simulink model "Optical_Movement_Detection_PAR"  (Simulink 7.5)
settings: Solver=ode45  StartTime=0.0  StopTime=inf  RelTol=1e-3
values from neighbouring files (symbols this model uses):
  D = 1    [Copter_Animation.m]
undefined symbols (not defined in the file or in its folder): Bottom, fspecial, Low, Rec, SDTV, sigbuilder_block
libraries: simulink x10, dspobslib x5, vipgeotforms x3, dspmtrx3 x2, vipanalysis x2, viptextngfix x2, vipsnks x2, dspsigops x2, vipconversions x1, dspswit3 x1, vipsrcs x1, dspstat3 x1
(part 2 of 2)

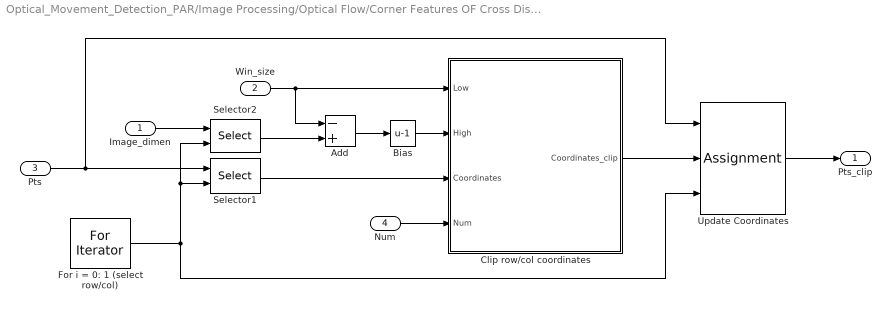
== system Optical_Movement_Detection_PAR/Image Processing/Optical Flow/Corner Features OF Cross Display/Corner Features OF/Corner Matching/Calculate Features/Clip Point Coordinates ==
  Image_dimen : Inport  OutDataType=sfix(16)  OutScaling=2^0
  Win_size : Inport  Port=2  OutDataType=sfix(16)  OutScaling=2^0
  Pts : Inport  Port=3
  Num : Inport  Port=4
  Add : Sum  Inputs=-+  OutDataType=sfix(16)  OutScaling=2^-10
  Bias : Bias  Bias=-1
  Clip row/col coordinates : Subsystem
  For i = 0: 1 (select row/col) : ForIterator  IterationLimit=2  IndexMode=Zero-based
  Selector1 : Selector  NumberOfDimensions=2  IndexMode=Zero-based  InputPortWidth=3  IndexOptions=Index vector (port),Select all  Indices=[1 3],1  OutputSizes=9,9
  Selector2 : Selector  IndexMode=Zero-based  InputPortWidth=2  IndexOptions=Index vector (port)  Indices=[1 3]  OutputSizes=9
  Update Coordinates : Assignment  NumberOfDimensions=2  IndexMode=Zero-based  IndexOptions=Index vector (port),Assign all  Indices=1,1  OutputSizes=81,50
  Pts_clip : Outport  OutDataType=sfix(16)  OutScaling=2^0
  wires:
  Selector2/1 -> Add/2
  For i = 0: 1 (select row/col)/1 -> Selector1/2, Selector2/2, Update Coordinates/3
  Clip row/col coordinates/1(Coordinates_clip) -> Update Coordinates/2
  Bias/1 -> Clip row/col coordinates/2(High)
  Update Coordinates/1 -> Pts_clip/1
  Num/1 -> Clip row/col coordinates/4(Num)
  Selector1/1 -> Clip row/col coordinates/3(Coordinates)
  Win_size/1 -> Add/1, Clip row/col coordinates/1(Low)
  Add/1 -> Bias/1
  Image_dimen/1 -> Selector2/1
  Pts/1 -> Update Coordinates/1, Selector1/1

== system Optical_Movement_Detection_PAR/Image Processing/Optical Flow/Corner Features OF Cross Display/Corner Features OF/Corner Matching/Calculate Distances/For Iterator Subsystem/For Iterator Subsystem ==
  F1 : Inport  OutDataType=sfix(16)  OutScaling=2^0
  N1 : Inport  Port=2  OutDataType=sfix(16)  OutScaling=2^0
  f2 : Inport  Port=3  OutDataType=sfix(16)  OutScaling=2^0
  Distance between two feature vectors : Subsystem
  For Iterator : ForIterator  IterationSource=external  IndexMode=Zero-based
  Select feature  for 1 corner : Selector  NumberOfDimensions=2  IndexMode=Zero-based  InputPortWidth=2  IndexOptions=Select all,Index vector (port)  Indices=0,1  OutputSizes=1,1
  Update feature  for a corner : Assignment  NumberOfDimensions=2  IndexMode=Zero-based  OutputInitialize=Specify size for each dimension in table  IndexOptions=Index vector (port),Assign all  Indices=1,1  OutputSizes=maxNum,1
  Dis : Outport  OutDataType=sfix(16)  OutScaling=2^0
  wires:
  Select feature  for 1 corner/1 -> Distance between two feature vectors/1(f1)
  f2/1 -> Distance between two feature vectors/2(f2)
  Update feature  for a corner/1 -> Dis/1
  F1/1 -> Select feature  for 1 corner/1
  For Iterator/1 -> Select feature  for 1 corner/2, Update feature  for a corner/2
  N1/1 -> For Iterator/1
  Distance between two feature vectors/1(dis) -> Update feature  for a corner/1

== system Optical_Movement_Detection_PAR/Image Processing/Optical Flow/Corner Features OF Cross Display/Corner Features OF/Corner Matching/Calculate Features/Clip Point Coordinates/Clip row/col coordinates ==
  Low : Inport  OutDataType=sfix(16)  OutScaling=2^0
  High : Inport  Port=2  OutDataType=sfix(16)  OutScaling=2^0
  Coordinates : Inport  Port=3
  Num : Inport  Port=4  OutDataType=sfix(16)  OutScaling=2^0
  Clip a Coordinate : Subsystem
  For Iterator : ForIterator  IterationSource=external  IterationLimit=2  IndexMode=Zero-based
  Select Coordinate of a Point : Selector  NumberOfDimensions=2  IndexMode=Zero-based  InputPortWidth=3  IndexOptions=Select all,Index vector (port)  Indices=[1 3],1  OutputSizes=9,1
  Update Feature  for a Corner : Assignment  NumberOfDimensions=2  IndexMode=Zero-based  IndexOptions=Assign all,Index vector (port)  Indices=1,1  OutputSizes=81,50
  Coordinates_clip : Outport  OutDataType=sfix(16)  OutScaling=2^0
  wires:
  Clip a Coordinate/1(Coordinate_clip) -> Update Feature  for a Corner/2
  Update Feature  for a Corner/1 -> Coordinates_clip/1
  High/1 -> Clip a Coordinate/2(High)
  Low/1 -> Clip a Coordinate/1(Low)
  Select Coordinate of a Point/1 -> Clip a Coordinate/3(Coordinate)
  Num/1 -> For Iterator/1
  Coordinates/1 -> Update Feature  for a Corner/1, Select Coordinate of a Point/1
  For Iterator/1 -> Select Coordinate of a Point/2, Update Feature  for a Corner/3

== system Optical_Movement_Detection_PAR/Image Processing/Optical Flow/Corner Features OF Cross Display/Corner Features OF/Corner Matching/Calculate Distances/For Iterator Subsystem/For Iterator Subsystem/Distance between two feature vectors ==
  f1 : Inport  OutDataType=sfix(16)  OutScaling=2^0
  f2 : Inport  Port=2  OutDataType=sfix(16)  OutScaling=2^0
  Abs : Abs  OutDataType=sfix(16)  OutScaling=2^0
  Add : Sum  Inputs=+-  OutDataType=sfix(16)  OutScaling=2^-10
  Sum of Elements : Sum  Inputs=+  OutDataType=sfix(16)  OutScaling=2^-10
  dis : Outport  OutDataType=sfix(16)  OutScaling=2^0
  wires:
  Sum of Elements/1 -> dis/1
  Abs/1 -> Sum of Elements/1
  Add/1 -> Abs/1
  f2/1 -> Add/2
  f1/1 -> Add/1

== system Optical_Movement_Detection_PAR/Image Processing/Optical Flow/Corner Features OF Cross Display/Corner Features OF/Corner Matching/Calculate Features/Clip Point Coordinates/Clip row/col coordinates/Clip a Coordinate ==
  Low : Inport  OutDataType=sfix(16)  OutScaling=2^0
  High : Inport  Port=2  OutDataType=sfix(16)  OutScaling=2^0
  Coordinate : Inport  Port=3  OutDataType=sfix(16)  OutScaling=2^0
  MinMax1 : MinMax  Function=max  Inputs=2  OutDataType=sfix(16)  OutScaling=2^0
  MinMax2 : MinMax  Inputs=2  OutDataType=sfix(16)  OutScaling=2^0
  Coordinate_clip : Outport  OutDataType=sfix(16)  OutScaling=2^0
  wires:
  MinMax2/1 -> Coordinate_clip/1
  High/1 -> MinMax2/2
  MinMax1/1 -> MinMax2/1
  Low/1 -> MinMax1/2
  Coordinate/1 -> MinMax1/1

== matlab function Image Processing/Optical Flow/Block Matching OF Cross Display/Optical Flow Segmentation in Sectors/Optical Flow Lines1 ==
  data: vel_Values input double; Cam_Img_Dim input double; vel_Lines output double; Omega_avg output double; scaleFactor parameter double size=1
function [vel_Lines, Omega_avg]=OpticalFlowLines(vel_Values, Cam_Img_Dim,scaleFactor) 

% Generates the coordinate points of optical flow lines

persistent first_time;
persistent X;
persistent Y;
persistent RV;
persistent CV;

%persistent Max_Vec_Length;

persistent Origin_Re;
persistent Origin_Im;

persistent Sec_1_Cnt;
persistent Sec_2_Cnt;
persistent Sec_3_Cnt;
persistent Sec_4_Cnt;

persistent Sec_1;
persistent Sec_2;
persistent Sec_3;
persistent Sec_4;

persistent R;
persistent C;
persistent Test_mat;
persistent med_vel_val;

%med_vel_val=median(vel_Values);
%[R C] = size(med_vel_val);
if isempty(first_time)
    first_time     = 1;
    Origin_Re = Cam_Img_Dim(1)/2%double(176);
    [R C] = size(vel_Values)
    Origin_Im = Cam_Img_Dim(2)/2%double(144);
end

Sec_1 = double(0);
Sec_2 = double(0);
Sec_3 = double(0);
Sec_4 = double(0);

Sec_1_Cnt = 1;
Sec_2_Cnt = 1;
Sec_3_Cnt = 1;
Sec_4_Cnt = 1;

%sectors
%       ^Im
%       |         
%   4   |  1
%-------------->Re
%   3   |  2
%       |

% for i=1:R
%     for k=1:C
%       j=vel_Values(i,k);
%     if(real(j)>=0) % Sec_1 or Sec_2
%         if(imag(j)>=0) %Sec_1
%             Sec_1_Cnt=Sec_1_Cnt+1;
%             Sec_1=Sec_1+double(abs(j))
%         else           %Sec_2
%             Sec_2_Cnt=Sec_2_Cnt+1;
%             Sec_2=Sec_2+double(abs(j))
%         end
%     else            % Sec_3 or Sec_4
%         if(imag(j)>=0) %Sec_4
%             Sec_4_Cnt=Sec_4_Cnt+1;
%             Sec_4=Sec_4+double(abs(j))
%         else           %Sec_3
%             Sec_3_Cnt=Sec_3_Cnt+1;
%             Sec_3=Sec_3+double(abs(j))
%         end
%     end
%     end
% end

%Other segm
for i=1:R
    for k=1:C
      j=vel_Values(i,k);
    if(real(j)>=0) % Sec_1 or Sec_2
        Sec_1_Cnt=Sec_1_Cnt+1;
        Sec_1=Sec_1+double(abs(real(j)));
        if(imag(j)>=0) %Sec_2
            Sec_2_Cnt=Sec_2_Cnt+1;
            Sec_2=Sec_2+double(imag(j));
        else           %Sec_4
            Sec_4_Cnt=Sec_4_Cnt+1;
            Sec_4=Sec_4+double(imag(j));
        end
    else            % Sec_3 or Sec_4
        Sec_3_Cnt=Sec_3_Cnt+1;
        Sec_3=Sec_3+double(abs(real(j)));
        if(imag(j)>=0) %Sec_2
            Sec_2_Cnt=Sec_2_Cnt+1;
            Sec_2=Sec_2+double(imag(j));
        else           %Sec_4
            Sec_4_Cnt=Sec_4_Cnt+1;
            Sec_4=Sec_4+double(imag(j));
        end
    end
    end
end


% Sec_1_Mat = vel_Values((real(vel_Values) >= 0) & (imag(vel_Values) >= 0));
% Sec_2_Mat = vel_Values((real(vel_Values) >= 0) & (imag(vel_Values) < 0));
% Sec_3_Mat = vel_Values((real(vel_Values) < 0) & (imag(vel_Values) < 0));
% Sec_4_Mat = vel_Values((real(vel_Values) < 0) & (imag(vel_Values) >= 0));


% Sec_1 = sum(abs(Sec_1_Mat)/(size(Sec_1_Mat, 1)*size(Sec_1_Mat, 2)));
% Sec_2 = sum(abs(Sec_1_Mat)/(size(Sec_1_Mat, 1)*size(Sec_1_Mat, 2)));
% Sec_3 = sum(abs(Sec_1_Mat)/(size(Sec_1_Mat, 1)*size(Sec_1_Mat, 2)));
% Sec_4 = sum(abs(Sec_1_Mat)/(size(Sec_1_Mat, 1)*size(Sec_1_Mat, 2)));

Sec_1 = Sec_1/Sec_1_Cnt;
Sec_2 = Sec_2/Sec_2_Cnt;
Sec_3 = Sec_3/Sec_3_Cnt;
Sec_4 = Sec_4/Sec_4_Cnt;

% Omega_Re_Plus = (scaleFactor*(Sec_1+Sec_2))/2
% Omega_Re_Minus = (scaleFactor*(Sec_3+Sec_4))/2
% Omega_Im_Plus = (scaleFactor*(Sec_1+Sec_4))/2
% Omega_Im_Minus = (scaleFactor*(Sec_3+Sec_2))/2

Omega_Re_Plus = scaleFactor*Sec_1; %Sec_2
Omega_Re_Minus = scaleFactor*Sec_3; %Sec_4
Omega_Im_Plus = scaleFactor*Sec_4; %Sec_1
Omega_Im_Minus = scaleFactor*Sec_2; %Sec_3

%Calculation of rotation

rotation_comp=min([abs(Omega_Re_Plus) abs(Omega_Re_Minus) abs(Omega_Im_Plus) abs(Omega_Im_Minus)]);

if(rotation_comp>0)
    Omega_avg = [abs(Omega_Re_Plus)-rotation_comp abs(Omega_Re_Minus)-rotation_comp abs(Omega_Im_Plus)-rotation_comp abs(Omega_Im_Minus)-rotation_comp rotation_comp];
else
    Omega_avg = [abs(Omega_Re_Plus) abs(Omega_Re_Minus) abs(Omega_Im_Plus) abs(Omega_Im_Minus) rotation_comp];
end


vel_Lines = [[Origin_Im Origin_Im Origin_Im Origin_Im];[Origin_Re Origin_Re Origin_Re Origin_Re];...
[Origin_Im Origin_Im+abs(Omega_Im_Minus) Origin_Im Origin_Im-abs(Omega_Im_Plus)];[Origin_Re+abs(Omega_Re_Plus) Origin_Re Origin_Re-abs(Omega_Re_Minus) Origin_Re]];

== matlab function Image Processing/Optical Flow/Cross for callibration/Optical Flow Lines1 ==
  data: vel_Values input double; Cam_Img_Dim input double; vel_Lines output double
function vel_Lines =OpticalFlowLines(vel_Values, Cam_Img_Dim) 

% Generates the coordinate points of optical flow lines

persistent first_time;
persistent X;
persistent Y;
persistent RV;
persistent CV;

%persistent Max_Vec_Length;

persistent Origin_Re;
persistent Origin_Im;

persistent Sec_1_Cnt;
persistent Sec_2_Cnt;
persistent Sec_3_Cnt;
persistent Sec_4_Cnt;

persistent Sec_1;
persistent Sec_2;
persistent Sec_3;
persistent Sec_4;

persistent R;
persistent C;
persistent Test_mat;
persistent med_vel_val;

%med_vel_val=median(vel_Values);
%[R C] = size(med_vel_val);
if isempty(first_time)
    first_time     = 1;
    Origin_Re = Cam_Img_Dim(1)/2%double(176);
    [R C] = size(vel_Values)
    Origin_Im = Cam_Img_Dim(2)/2%double(144);
end


Omega_Re_Plus = 700;
Omega_Re_Minus = 700;
Omega_Im_Plus = 700;
Omega_Im_Minus = 700;


vel_Lines = [[Origin_Im Origin_Im Origin_Im Origin_Im];[Origin_Re Origin_Re Origin_Re Origin_Re];...
[Origin_Im Origin_Im+abs(Omega_Im_Minus) Origin_Im Origin_Im-abs(Omega_Im_Plus)];[Origin_Re+abs(Omega_Re_Plus) Origin_Re Origin_Re-abs(Omega_Re_Minus) Origin_Re]];

== matlab function Image Processing/Optical Flow/Corner Features OF Cross Display/Corner Features OF/Embedded MATLAB Function ==
  data: vec output double; Tform input double; allowNewCalc input double; rot output double; TsOpt input double
function [vec, rot] = clc(Tform, allowNewCalc, TsOpt)
%#eml
persistent vec_old;
persistent rot_old;
persistent first_time;
persistent db_3_filter;

if isempty(first_time)
    vec_old = double(complex(0,0));
    vec = double(complex(0,0));
    rot = double(0);
    rot_old = double(0);
    first_time=1;
    db_3_filter=double([0;0;0;0;0;0;0]);
end
    Tform
    %v'=Tform*v with v=[x y 1]^T and v'=[x' y' 1]
    if(allowNewCalc)
    vec=double(complex(Tform(2,3),Tform(1,3)));
    rot=double(abs(-asin(complex(Tform(1,2)))))/TsOpt;
    %Detect direction of rotation
    if((Tform(1,3) > 0) && Tform(2,3) < 0)
        %counterclockwise is negative
        rot=rot*(-1);
    end
    db_3_filter=circshift(db_3_filter, 1);
    db_3_filter(1,1)=rot;
    db_3_filter
    rot=sum(db_3_filter)/7;
    vec_old=vec;
    rot_old=rot;
else
vec=vec_old;
rot=rot_old;
end

== matlab function Image Processing/Optical Flow/Corner Features OF Cross Display/Optical Flow Segmentation in Sectors Corner Features/Optical Flow Lines1 ==
  data: vel_Values input double; Cam_Img_Dim input double; rotation input double; vel_Lines output double; Omega_avg output double; scaleFactor parameter double size=1
function [vel_Lines, Omega_avg]=OpticalFlowLines(vel_Values, Cam_Img_Dim, rotation ,scaleFactor) 

% Generates the coordinate points of optical flow lines

persistent first_time;
persistent X;
persistent Y;
persistent RV;
persistent CV;

%persistent Max_Vec_Length;

persistent Origin_Re;
persistent Origin_Im;

persistent Sec_1_Cnt;
persistent Sec_2_Cnt;
persistent Sec_3_Cnt;
persistent Sec_4_Cnt;

persistent Sec_1;
persistent Sec_2;
persistent Sec_3;
persistent Sec_4;

persistent R;
persistent C;
persistent Test_mat;
persistent med_vel_val;

%med_vel_val=median(vel_Values);
%[R C] = size(med_vel_val);
if isempty(first_time)
    first_time     = 1;
    Origin_Re = Cam_Img_Dim(1)/2%double(176);
    [R C] = size(vel_Values)
    Origin_Im = Cam_Img_Dim(2)/2%double(144);
end

Sec_1 = double(0);
Sec_2 = double(0);
Sec_3 = double(0);
Sec_4 = double(0);

Sec_1_Cnt = 1;
Sec_2_Cnt = 1;
Sec_3_Cnt = 1;
Sec_4_Cnt = 1;

%sectors
%       ^Im
%       |         
%   4   |  1
%-------------->Re
%   3   |  2
%       |

% for i=1:R
%     for k=1:C
%       j=vel_Values(i,k);
%     if(real(j)>=0) % Sec_1 or Sec_2
%         if(imag(j)>=0) %Sec_1
%             Sec_1_Cnt=Sec_1_Cnt+1;
%             Sec_1=Sec_1+double(abs(j))
%         else           %Sec_2
%             Sec_2_Cnt=Sec_2_Cnt+1;
%             Sec_2=Sec_2+double(abs(j))
%         end
%     else            % Sec_3 or Sec_4
%         if(imag(j)>=0) %Sec_4
%             Sec_4_Cnt=Sec_4_Cnt+1;
%             Sec_4=Sec_4+double(abs(j))
%         else           %Sec_3
%             Sec_3_Cnt=Sec_3_Cnt+1;
%             Sec_3=Sec_3+double(abs(j))
%         end
%     end
%     end
% end

%Other segm
for i=1:R
    for k=1:C
      j=vel_Values(i,k);
    if(real(j)>=0) % Sec_1 or Sec_2
        Sec_1_Cnt=Sec_1_Cnt+1;
        Sec_1=Sec_1+double(abs(real(j)));
        if(imag(j)>=0) %Sec_2
            Sec_2_Cnt=Sec_2_Cnt+1;
            Sec_2=Sec_2+double(imag(j));
        else           %Sec_4
            Sec_4_Cnt=Sec_4_Cnt+1;
            Sec_4=Sec_4+double(imag(j));
        end
    else            % Sec_3 or Sec_4
        Sec_3_Cnt=Sec_3_Cnt+1;
        Sec_3=Sec_3+double(abs(real(j)));
        if(imag(j)>=0) %Sec_2
            Sec_2_Cnt=Sec_2_Cnt+1;
            Sec_2=Sec_2+double(imag(j));
        else           %Sec_4
            Sec_4_Cnt=Sec_4_Cnt+1;
            Sec_4=Sec_4+double(imag(j));
        end
    end
    end
end


% Sec_1_Mat = vel_Values((real(vel_Values) >= 0) & (imag(vel_Values) >= 0));
% Sec_2_Mat = vel_Values((real(vel_Values) >= 0) & (imag(vel_Values) < 0));
% Sec_3_Mat = vel_Values((real(vel_Values) < 0) & (imag(vel_Values) < 0));
% Sec_4_Mat = vel_Values((real(vel_Values) < 0) & (imag(vel_Values) >= 0));


% Sec_1 = sum(abs(Sec_1_Mat)/(size(Sec_1_Mat, 1)*size(Sec_1_Mat, 2)));
% Sec_2 = sum(abs(Sec_1_Mat)/(size(Sec_1_Mat, 1)*size(Sec_1_Mat, 2)));
% Sec_3 = sum(abs(Sec_1_Mat)/(size(Sec_1_Mat, 1)*size(Sec_1_Mat, 2)));
% Sec_4 = sum(abs(Sec_1_Mat)/(size(Sec_1_Mat, 1)*size(Sec_1_Mat, 2)));

Sec_1 = Sec_1/Sec_1_Cnt;
Sec_2 = Sec_2/Sec_2_Cnt;
Sec_3 = Sec_3/Sec_3_Cnt;
Sec_4 = Sec_4/Sec_4_Cnt;

% Omega_Re_Plus = (scaleFactor*(Sec_1+Sec_2))/2
% Omega_Re_Minus = (scaleFactor*(Sec_3+Sec_4))/2
% Omega_Im_Plus = (scaleFactor*(Sec_1+Sec_4))/2
% Omega_Im_Minus = (scaleFactor*(Sec_3+Sec_2))/2

Omega_Re_Plus = scaleFactor*Sec_1; %Sec_2
Omega_Re_Minus = scaleFactor*Sec_3; %Sec_4
Omega_Im_Plus = scaleFactor*Sec_4; %Sec_1
Omega_Im_Minus = scaleFactor*Sec_2; %Sec_3

%Calculation of rotation

rotation_comp=scaleFactor*rotation;;

if(rotation_comp>0)
    Omega_avg = [abs(Omega_Re_Plus)-rotation_comp abs(Omega_Re_Minus)-rotation_comp abs(Omega_Im_Plus)-rotation_comp abs(Omega_Im_Minus)-rotation_comp rotation_comp];
else
    Omega_avg = [abs(Omega_Re_Plus) abs(Omega_Re_Minus) abs(Omega_Im_Plus) abs(Omega_Im_Minus) rotation_comp];
end


vel_Lines = [[Origin_Im Origin_Im Origin_Im Origin_Im];[Origin_Re Origin_Re Origin_Re Origin_Re];...
[Origin_Im Origin_Im+abs(Omega_Im_Minus) Origin_Im Origin_Im-abs(Omega_Im_Plus)];[Origin_Re+abs(Omega_Re_Plus) Origin_Re Origin_Re-abs(Omega_Re_Minus) Origin_Re]];
